simulink model "task2e_2015"  (R2015a)
settings: Solver=ode45  SolverMode=SingleTasking  StartTime=0.0  StopTime=10.0  RelTol=1e-3
values from neighbouring files (symbols this model uses):
  g = 9.8    [task1.m]    (also in task2c.m; task2e.m = 9.81; task2f.m = 9.81)
  l = l_hat_linf    [task1.m]    (also in task2c.m = 0.3; task2e.m = 0.3; task2f.m = 0.3)
  V = linf.V    [task2e.m]    (also in task2f.m)
undefined symbols (not defined in the file or in its folder): k1, ms, mw
settings Model: CovMetricSettings=dwe  CovHtmlReporting=off  covSaveCumulativeToWorkspaceVar=off  CovSaveSingleToWorkspaceVar=off  CovExternalEMLEnable=on  Creator=NicSch02  LastModifiedBy=NicSch02
settings DataIOCC: LimitDataPoints=off  SaveFormat=Dataset  ReturnWorkspaceOutputs=on
settings DebuggingCC: SFUnexpectedBacktrackingDiag=error  SFNoUnconditionalDefaultTransitionDiag=error
settings HardwareCC: ProdBitPerPointer=64  ProdLargestAtomicFloat=Float  ProdIntDivRoundTo=Zero  ProdEndianess=LittleEndian  ProdHWDeviceType=Specified
settings ModelReferenceCC: PropagateSignalLabelsOutOfModel=on
settings SFSimCC: SimUseLocalCustomCode=on
settings RTWCC: RTWUseLocalCustomCode=on
settings GRTTargetCC: TargetLangStandard=C99 (ISO)  GeneratePreprocessorConditionals=Use local settings

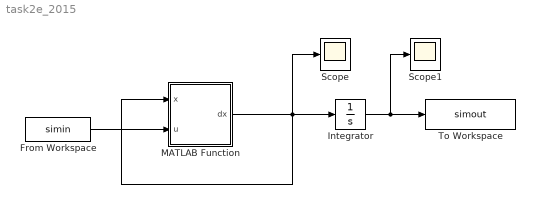
== system task2e_2015 ==
  From Workspace : FromWorkspace  VariableName=simin  SampleTime=0
  Integrator : Integrator
  MATLAB Function : MATLAB Function  TreatAsAtomicUnit=on
      settings: PermitHierarchicalResolution=ParametersOnly
  Scope : Scope
      settings: TimeRange=auto  MaxDataPoints=5000  SaveToWorkspace=off  SaveName=ScopeData  YMin=-10  YMax=10  SampleTime=-1
  Scope1 : Scope
      settings: TimeRange=auto  MaxDataPoints=5000  SaveToWorkspace=off  YMin=-10  YMax=10  SampleTime=-1
  To Workspace : ToWorkspace  VariableName=simout  SaveFormat=Timeseries  SampleTime=-1
  wires:
  MATLAB Function/1(dx) -> Scope/1, MATLAB Function/1(x), Integrator/1
  Integrator/1 -> Scope1/1, To Workspace/1
  From Workspace/1 -> MATLAB Function/2(u)

== matlab function task2e_2015/MATLAB Function ==
  data: x input; g parameter; dx output; l parameter; u input; ms parameter; mw parameter; V parameter; k1 parameter
function dx = fcn(x,g,l,u, ms, mw, V, k1)
dx = [0;0;0;0];

dx(1) = x(3);
dx(2) = x(4);
dx(3) = (1/(mw+ms(1-cos(x(2))^2)))*(V*u - k1*x(3) + ms*l*x(4)^2*sin(x(2)) - ms*g*sin(x(2))*cos(x(2)));
dx(4) = (1/(1-(ms/(mw+ms))*cos(x(2))^2))*(g*sin(x(2)) - (cos(x(2))/(mw+ms))*(V*u-k1*x(3)) - ((ms/(mw+ms))*l*x(4)^2)*sin(x(2))*cos(x(2)));
